simulink model "Copter_sf"  (R2012b)
settings: Solver=FixedStepDiscrete  StartTime=0.0  StopTime=inf  FixedStep=T_sim  MaxStep=0.01  RelTol=1e-5
settings Model: Creator=David  LastModifiedBy=David
settings DataIOCC: ExternalInput=getinputstruct(op_trim1)  InitialState=getstatestruct(op_trim1)  SaveFormat=Structure  SaveOutput=off  SaveTime=off  Refine=10
settings OptimizationCC: InlineParams=on
settings DebuggingCC: UnderspecifiedInitializationDetection=Simplified  MergeDetectMultiDrivingBlocksExec=error  CheckMatrixSingularityMsg=warning  IntegerOverflowMsg=error  Int32ToFloatConvMsg=none  ParameterUnderflowMsg=error  UnderSpecifiedDataTypeMsg=warning  AssertControl=DisableAll
settings HardwareCC: ProdBitPerLong=64

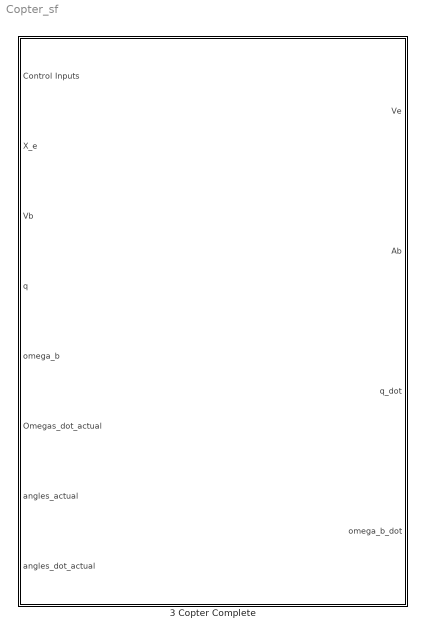
== system Copter_sf ==
  3 Copter Complete : Subsystem
      mask help: Simulink:masks:GenSFuncDesc_MD
      mask Help: eval('feval(''rtwprivate'',''rtwhelpview'',''rtw_sfcn_block'')');

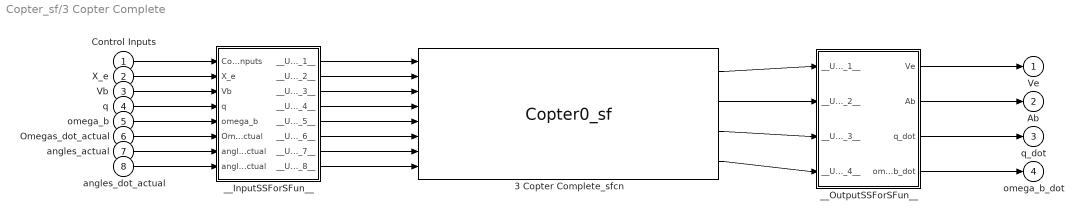
== system Copter_sf/3 Copter Complete ==
  Control Inputs : Inport
  X_e : Inport  Port=2
  Vb : Inport  Port=3
  q : Inport  Port=4
  omega_b : Inport  Port=5
  Omegas_dot_actual : Inport  Port=6
  angles_actual : Inport  Port=7
  angles_dot_actual : Inport  Port=8
  3 Copter Complete_sfcn : S-Function  FunctionName=Copter0_sf  SFunctionModules=""  EnableBusSupport=off  mask{rtw_sf_name=Copter0_sf, showVar=off}
      mask prompts: rtw_sf_name "Simulink:masks:GenSFuncName_MP"; showVar "Simulink:masks:GenSFuncShowModuleList_MP"
      mask help: Simulink:masks:GenSFuncDesc_MD
      mask init:
      | displist = '';
      | if ~strcmp(get_param(gcb, 'FunctionName'), rtw_sf_name);
      |   set_param(gcb, 'FunctionName', rtw_sf_name);
      | end
      | % Check if we are generating code
      | rtw_mode = false;
      | if strcmpi(get_param(bdroot(gcb),'SimulationStatus'),'Initializing')
      | 	rtw_mode = strcmpi(get_param(bdroot(gcb),'BuildingRTWCode'),'on') && ...
      | 		~strcmpi(get_param(bdroot(gcb),'TargetStyle'),'SimulationTarget');
      | end
      | if showVar || rtw_mode
      | 	if exist('rtwsfunc') == 2 | exist('rtwsfunc') == 6
      | 		tmplist = rtwsfunc(rtw_sf_name,gcb);
      | 		tmplist = DAStudio.message('Simulink:masks:GenSFuncListOfModules_IC', tmplist);
      | 	elseif showVar
      | 		tmplist1 = DAStudio.message('Simulink:masks:GenSFuncListOfModules_IC', '');
      |         tmplist2 = DAStudio.message('Simulink:masks:GenSFuncNotLicensed_IC');
      |         tmplist = [tmplist1 tmplist2];
      |  	end
      | end
      | if showVar
      |   displist = tmplist;
      | end
      settings: CopyFcn=|
      | if ~strcmp(get_param(gcb,'Linkstatus'),'none') && ...
      | ~strcmp(get_param(gcb,'Linkstatus'),'implicit')
      |   set_param(gcb,'LinkStatus','none');
      | end
      mask Help: eval('feval(''rtwprivate'',''rtwhelpview'',''rtw_sfcn_block'')');
      mask Display:
      | port_label('input',1,'Control Inputs');
      | port_label('input',2,'X_e');
      | port_label('input',3,'Vb');
      | port_label('input',4,'q');
      | port_label('input',5,'omega_b');
      | port_label('input',6,'Omegas_dot_actual');
      | port_label('input',7,'angles_actual');
      | port_label('input',8,'angles_dot_actual');
      | port_label('output',1,'Ve');
      | port_label('output',2,'Ab');
      | port_label('output',3,'q_dot');
      | port_label('output',4,'omega_b_dot');
  __InputSSForSFun__ : Subsystem
  __OutputSSForSFun__ : Subsystem
  Ve : Outport
  Ab : Outport  Port=2
  q_dot : Outport  Port=3
  omega_b_dot : Outport  Port=4
  wires:
  Control Inputs/1 -> __InputSSForSFun__/1(Control Inputs)
  X_e/1 -> __InputSSForSFun__/2(X_e)
  Vb/1 -> __InputSSForSFun__/3(Vb)
  q/1 -> __InputSSForSFun__/4(q)
  omega_b/1 -> __InputSSForSFun__/5(omega_b)
  Omegas_dot_actual/1 -> __InputSSForSFun__/6(Omegas_dot_actual)
  angles_actual/1 -> __InputSSForSFun__/7(angles_actual)
  angles_dot_actual/1 -> __InputSSForSFun__/8(angles_dot_actual)
  __InputSSForSFun__/1(__UniqueOutportName__1__) -> 3 Copter Complete_sfcn/1
  __InputSSForSFun__/2(__UniqueOutportName__2__) -> 3 Copter Complete_sfcn/2
  __InputSSForSFun__/3(__UniqueOutportName__3__) -> 3 Copter Complete_sfcn/3
  __InputSSForSFun__/4(__UniqueOutportName__4__) -> 3 Copter Complete_sfcn/4
  __InputSSForSFun__/5(__UniqueOutportName__5__) -> 3 Copter Complete_sfcn/5
  __InputSSForSFun__/6(__UniqueOutportName__6__) -> 3 Copter Complete_sfcn/6
  __InputSSForSFun__/7(__UniqueOutportName__7__) -> 3 Copter Complete_sfcn/7
  __InputSSForSFun__/8(__UniqueOutportName__8__) -> 3 Copter Complete_sfcn/8
  3 Copter Complete_sfcn/1 -> __OutputSSForSFun__/1(__UniqueInportName__1__)
  3 Copter Complete_sfcn/2 -> __OutputSSForSFun__/2(__UniqueInportName__2__)
  3 Copter Complete_sfcn/3 -> __OutputSSForSFun__/3(__UniqueInportName__3__)
  3 Copter Complete_sfcn/4 -> __OutputSSForSFun__/4(__UniqueInportName__4__)
  __OutputSSForSFun__/1(Ve) -> Ve/1
  __OutputSSForSFun__/2(Ab) -> Ab/1
  __OutputSSForSFun__/3(q_dot) -> q_dot/1
  __OutputSSForSFun__/4(omega_b_dot) -> omega_b_dot/1

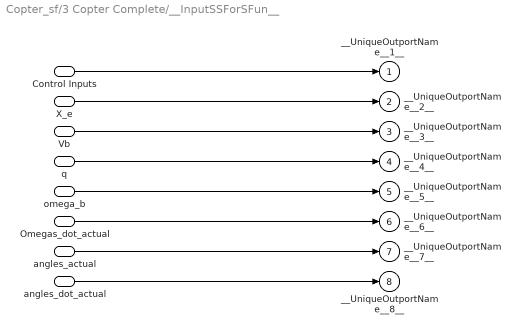
== system Copter_sf/3 Copter Complete/__InputSSForSFun__ ==
  Control Inputs : Inport
  X_e : Inport  Port=2
  Vb : Inport  Port=3
  q : Inport  Port=4
  omega_b : Inport  Port=5
  Omegas_dot_actual : Inport  Port=6
  angles_actual : Inport  Port=7
  angles_dot_actual : Inport  Port=8
  __UniqueOutportName__1__ : Outport
  __UniqueOutportName__2__ : Outport  Port=2
  __UniqueOutportName__3__ : Outport  Port=3
  __UniqueOutportName__4__ : Outport  Port=4
  __UniqueOutportName__5__ : Outport  Port=5
  __UniqueOutportName__6__ : Outport  Port=6
  __UniqueOutportName__7__ : Outport  Port=7
  __UniqueOutportName__8__ : Outport  Port=8
  wires:
  Control Inputs/1 -> __UniqueOutportName__1__/1
  X_e/1 -> __UniqueOutportName__2__/1
  Vb/1 -> __UniqueOutportName__3__/1
  q/1 -> __UniqueOutportName__4__/1
  omega_b/1 -> __UniqueOutportName__5__/1
  Omegas_dot_actual/1 -> __UniqueOutportName__6__/1
  angles_actual/1 -> __UniqueOutportName__7__/1
  angles_dot_actual/1 -> __UniqueOutportName__8__/1

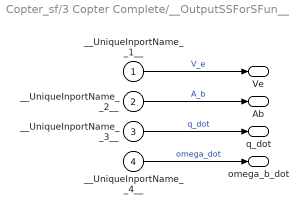
== system Copter_sf/3 Copter Complete/__OutputSSForSFun__ ==
  __UniqueInportName__1__ : Inport
  __UniqueInportName__2__ : Inport  Port=2
  __UniqueInportName__3__ : Inport  Port=3
  __UniqueInportName__4__ : Inport  Port=4
  Ve : Outport
  Ab : Outport  Port=2
  q_dot : Outport  Port=3
  omega_b_dot : Outport  Port=4
  wires:
  __UniqueInportName__1__/1 -> Ve/1  "V_e"
  __UniqueInportName__2__/1 -> Ab/1  "A_b"
  __UniqueInportName__3__/1 -> q_dot/1  "q_dot"
  __UniqueInportName__4__/1 -> omega_b_dot/1  "omega_dot"
